simulink model "ABS_discDyn_model"  (R2022b)
settings: Solver=VariableStepAuto  StartTime=0.0  StopTime=tf  MaxStep=1e-3  RelTol=1e-3  EnableMultiTasking=on
values from neighbouring files (symbols this model uses):
  init_speed = 100    [mainABS.m]
  lambda_max = 0.25    [mainABS.m]
  lambda_min = 0.08    [mainABS.m]
  omega_act = 70    [mainABS.m]
  tau_delay = 10e-3    (= 0.01)    [mainABS.m]
  Tb_max = 1400    [mainABS.m]
  Tb_min = 1150    [mainABS.m]
undefined symbols (not defined in the file or in its folder): auxdata
libraries: simulink x1
settings Model: Creator=luca  LastModifiedBy=giacomo
settings SolverCC: AlgebraicLoopSolver=TrustRegion
settings DataIOCC: LimitDataPoints=on  ReturnWorkspaceOutputs=off
settings OptimizationCC: LifeSpan=inf
settings DebuggingCC: UnconnectedInputMsg=warning  UnconnectedOutputMsg=warning  UnconnectedLineMsg=warning  AllowSymbolicDim=off  SFUnexpectedBacktrackingDiag=warning  SFNoUnconditionalDefaultTransitionDiag=warning  SFExecutionAtInitializationDiag=none  SFMachineParentedDataDiag=warning  ArithmeticOperatorsInVariantConditions=warning
settings ModelReferenceCC: EnableRefExpFcnMdlSchedulingChecks=on  PropagateSignalLabelsOutOfModel=off
settings SFSimCC: SimUseLocalCustomCode=off  CustomCodeUndefinedFunction=UseInterfaceOnly
settings RTWCC: RTWUseLocalCustomCode=off
settings CodeAppCC: StateflowObjectComments=on
settings GRTTargetCC: TargetLangStandard=C89/C90 (ANSI)
settings ConfigComp: CovMetricSettings=dw  CovSaveCumulativeToWorkspaceVar=on  CovSaveSingleToWorkspaceVar=on  CovExternalEMLEnable=off

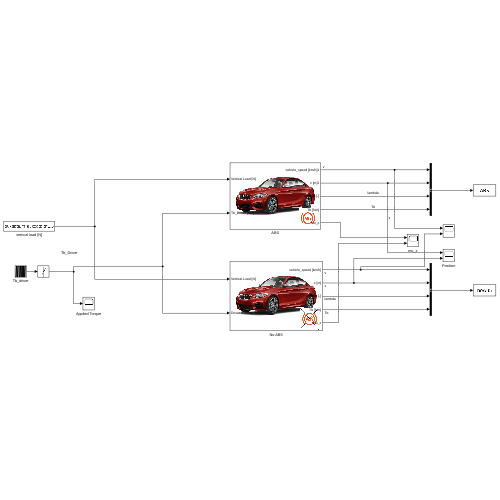
[thumbnail: Simulink's stored preview of the top-level diagram]
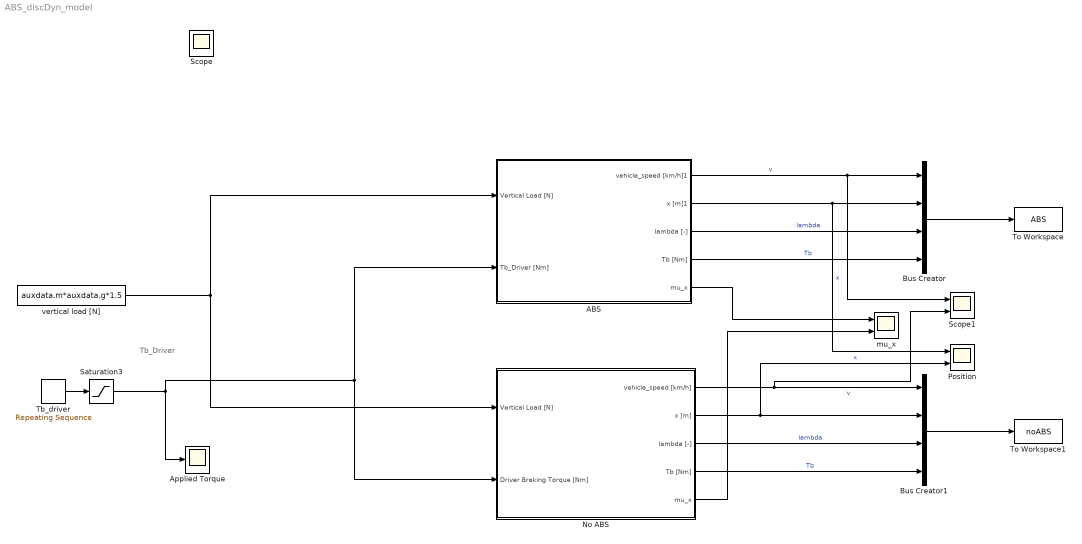
== system ABS_discDyn_model ==
  note: Tb_Driver
  ABS : Subsystem
      mask Display: image('figures/ABScar_on.png');
  Applied Torque : Scope
  Bus Creator : BusCreator  Inputs=4
  Bus Creator1 : BusCreator  Inputs=4
  No ABS : Subsystem
      mask Display: image('figures/ABS_off.png');
  Position : Scope  NumInputPorts=2
  Saturation3 : Saturate  UpperLimit=Tb_max  LowerLimit=0
  Scope1 : Scope  NumInputPorts=2
  Tb_driver : simulink/Sources/Repeating Sequence  rep_seq_t=time_manoeuvre  rep_seq_y=output_manoeuvre
  To Workspace : ToWorkspace  VariableName=ABS  SaveFormat=Timeseries  SampleTime=-1
  To Workspace1 : ToWorkspace  VariableName=noABS  SaveFormat=Timeseries  SampleTime=-1
  mu_x : Scope  NumInputPorts=2
  vertical load [N] : Constant  Value=auxdata.m*auxdata.g*1.5
  Scope : Scope
  wires:
  vertical load [N]/1 -> ABS/1(Vertical Load [N]), No ABS/1(Vertical Load [N])
  No ABS/1(" vehicle_speed [km/h]") -> Scope1/2, Bus Creator1/1  "v"
  No ABS/2(x [m]) -> Position/2, Bus Creator1/2  "x"
  ABS/1(vehicle_speed [km/h]1) -> Scope1/1, Bus Creator/1  "v"
  ABS/2(x [m]1) -> Position/1, Bus Creator/2  "x"
  Bus Creator/1 -> To Workspace/1
  ABS/3(lambda [-]) -> Bus Creator/3  "lambda"
  ABS/4(Tb [Nm]) -> Bus Creator/4  "Tb"
  Bus Creator1/1 -> To Workspace1/1
  No ABS/3(lambda [-]) -> Bus Creator1/3  "lambda"
  No ABS/4(Tb [Nm]) -> Bus Creator1/4  "Tb"
  Saturation3/1 -> ABS/2(Tb_Driver [Nm]), No ABS/2(Driver Braking Torque [Nm]), Applied Torque/1
  Tb_driver/1 -> Saturation3/1
  No ABS/5(mu_x) -> mu_x/2
  ABS/5(mu_x) -> mu_x/1

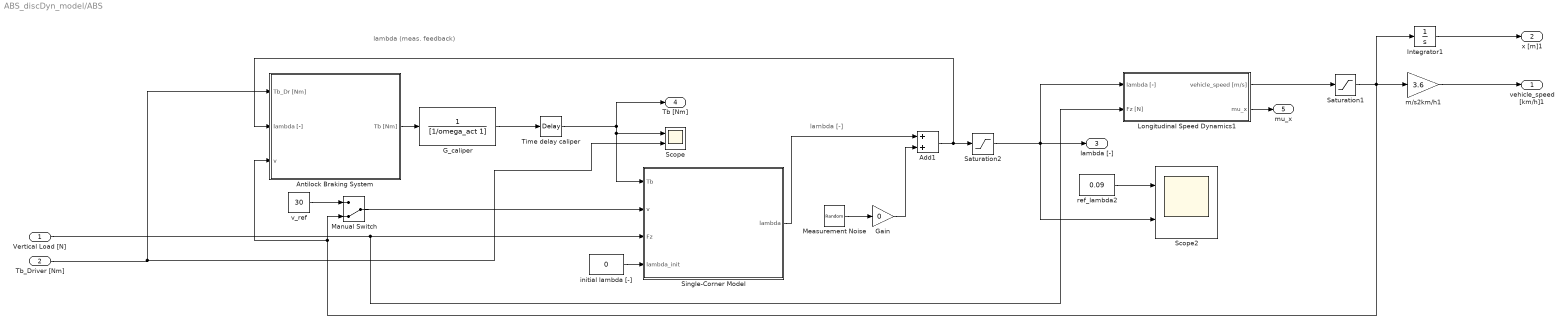
== system ABS_discDyn_model/ABS ==
  note: lambda (meas. feedback)
  note: lambda [-]
  Vertical Load [N] : Inport
  Tb_Driver [Nm] : Inport  Port=2
  Add1 : Sum
  Antilock Braking System : Subsystem
      mask Display: image('figures/ABS_on.png');
  G_caliper : TransferFcn  Numerator=1  Denominator=[1/omega_act 1]
  Gain : Gain  Gain=0
  Integrator1 : Integrator
  Longitudinal Speed Dynamics1 : Subsystem
  Manual Switch : ManualSwitch  CurrentSetting=0
  Measurement Noise : RandomNumber  Variance=2e-5  SampleTime=0.001
  Saturation1 : Saturate  UpperLimit=100  LowerLimit=1e-3
  Saturation2 : Saturate  UpperLimit=1  LowerLimit=0
  Scope : Scope  NumInputPorts=2
  Scope2 : Scope  NumInputPorts=2
  Single-Corner Model : Subsystem
      mask Display:
      | image('figures/caliper_img.jpeg');
      | color('red');
      | port_label('output',1,'lambda');
      | port_label('input',1,'Tb');
      | port_label('input',2,'v');
      | port_label('input',3,'Fz');
      | port_label('input',4,'lambda_init');
  Time delay caliper : TransportDelay  DelayTime=tau_delay
  initial lambda [-] : Constant  Value=0
  m/s2km/h1 : Gain  Gain=3.6
  ref_lambda2 : Constant  Value=0.09
  v_ref : Constant  Value=30
  vehicle_speed [km/h]1 : Outport
  x [m]1 : Outport  Port=2
  lambda [-] : Outport  Port=3
  Tb [Nm] : Outport  Port=4
  mu_x : Outport  Port=5
  wires:
  Add1/1 -> Antilock Braking System/2(lambda [-]), Saturation2/1
  m/s2km/h1/1 -> vehicle_speed [km/h]1/1
  Tb_Driver [Nm]/1 -> Antilock Braking System/1(Tb_Dr [Nm]), Scope/2
  Antilock Braking System/1(Tb [Nm]) -> G_caliper/1
  Saturation2/1 -> lambda [-]/1, Scope2/2, Longitudinal Speed Dynamics1/1(lambda [-])
  Gain/1 -> Add1/2
  initial lambda [-]/1 -> Single-Corner Model/4(lambda_init)
  Longitudinal Speed Dynamics1/1(vehicle_speed [m/s]) -> Saturation1/1
  Integrator1/1 -> x [m]1/1
  Single-Corner Model/1(lambda) -> Add1/1
  Vertical Load [N]/1 -> Single-Corner Model/3(Fz), Longitudinal Speed Dynamics1/2(Fz [N])
  ref_lambda2/1 -> Scope2/1
  Measurement Noise/1 -> Gain/1
  Saturation1/1 -> Antilock Braking System/3(v), Manual Switch/2, Integrator1/1, m/s2km/h1/1
  Manual Switch/1 -> Single-Corner Model/2(v)
  v_ref/1 -> Manual Switch/1
  Longitudinal Speed Dynamics1/2(mu_x) -> mu_x/1
  G_caliper/1 -> Time delay caliper/1
  Time delay caliper/1 -> Tb [Nm]/1, Single-Corner Model/1(Tb), Scope/1

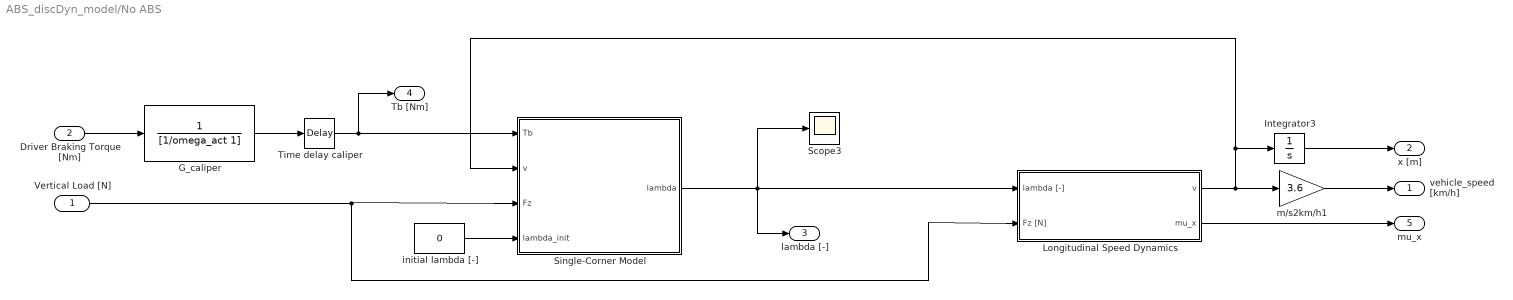
== system ABS_discDyn_model/No ABS ==
  Vertical Load [N] : Inport
  Driver Braking Torque [Nm] : Inport  Port=2
  G_caliper : TransferFcn  Numerator=1  Denominator=[1/omega_act 1]
  Integrator3 : Integrator
  Longitudinal Speed Dynamics : Subsystem
  Scope3 : Scope
  Single-Corner Model : Subsystem
      mask Display:
      | image('figures/caliper_img.jpeg');
      | color('red');
      | port_label('output',1,'lambda [-]');
      | port_label('input',1,'Tb [Nm]');
      | port_label('input',2,'v [m/s]');
      | port_label('input',3,'Fz [N]');
      | port_label('input',4,'lambda_init [-]');
  Time delay caliper : TransportDelay  DelayTime=tau_delay
  initial lambda [-] : Constant  Value=0
  m/s2km/h1 : Gain  Gain=3.6
  " vehicle_speed [km/h]" : Outport
  x [m] : Outport  Port=2
  lambda [-] : Outport  Port=3
  Tb [Nm] : Outport  Port=4
  mu_x : Outport  Port=5
  wires:
  Single-Corner Model/1(lambda) -> lambda [-]/1, Longitudinal Speed Dynamics/1(lambda [-]), Scope3/1
  Vertical Load [N]/1 -> Single-Corner Model/3(Fz), Longitudinal Speed Dynamics/2(Fz [N])
  Time delay caliper/1 -> Tb [Nm]/1, Single-Corner Model/1(Tb)
  initial lambda [-]/1 -> Single-Corner Model/4(lambda_init)
  m/s2km/h1/1 -> " vehicle_speed [km/h]"/1
  Integrator3/1 -> x [m]/1
  Longitudinal Speed Dynamics/1(v) -> Single-Corner Model/2(v), Integrator3/1, m/s2km/h1/1
  Longitudinal Speed Dynamics/2(mu_x) -> mu_x/1
  G_caliper/1 -> Time delay caliper/1
  Driver Braking Torque [Nm]/1 -> G_caliper/1

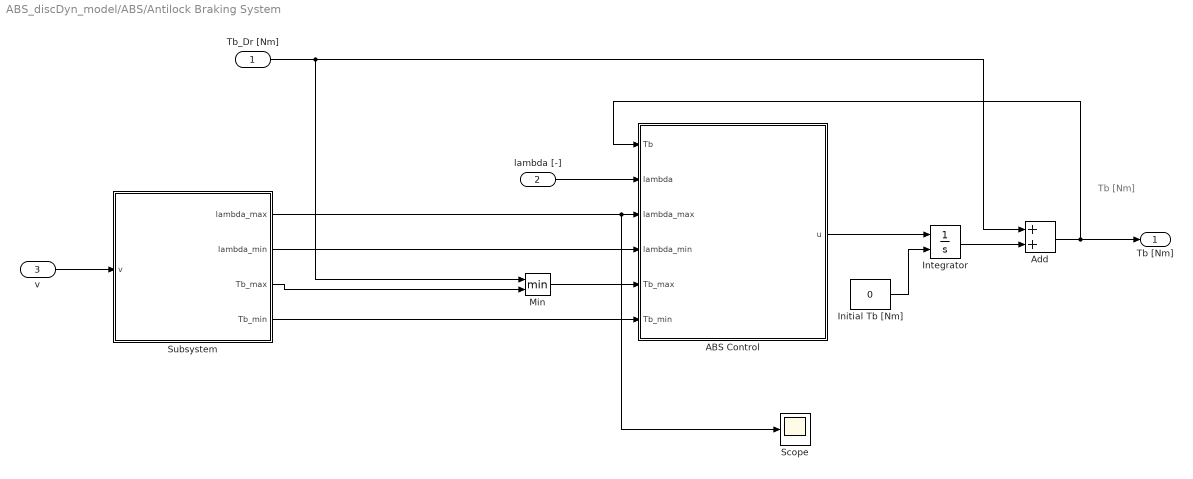
== system ABS_discDyn_model/ABS/Antilock Braking System ==
  note: Tb [Nm]
  Tb_Dr [Nm] : Inport
  lambda [-] : Inport  Port=2
  v : Inport  Port=3
  ABS Control : Stateflow chart  TreatAsAtomicUnit=on
  Add : Sum
  Initial Tb [Nm] : Constant  Value=0
  Integrator : Integrator  InitialConditionSource=external
  Min : MinMax  Inputs=2
  Scope : Scope
  Subsystem : Subsystem
  Tb [Nm] : Outport
  wires:
  lambda [-]/1 -> ABS Control/2(lambda)
  Initial Tb [Nm]/1 -> Integrator/2
  Add/1 -> ABS Control/1(Tb), Tb [Nm]/1
  ABS Control/1(u) -> Integrator/1
  Integrator/1 -> Add/2
  Tb_Dr [Nm]/1 -> Min/1, Add/1
  Subsystem/1(lambda_max) -> Scope/1, ABS Control/3(lambda_max)
  v/1 -> Subsystem/1(v)
  Subsystem/4(Tb_min) -> ABS Control/6(Tb_min)
  Subsystem/2(lambda_min) -> ABS Control/4(lambda_min)
  Min/1 -> ABS Control/5(Tb_max)
  Subsystem/3(Tb_max) -> Min/2

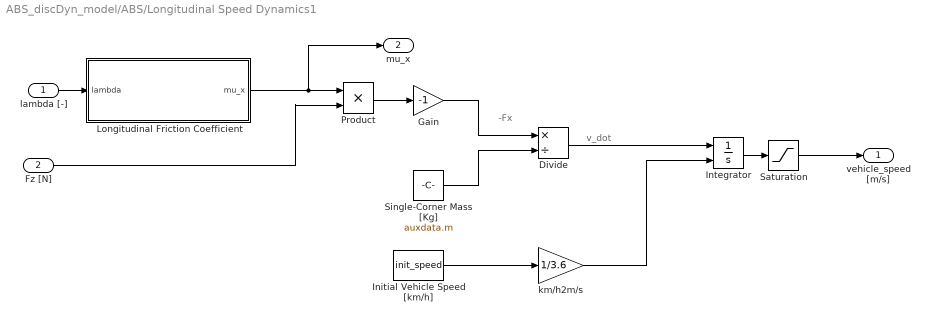
== system ABS_discDyn_model/ABS/Longitudinal Speed Dynamics1 ==
  note: -Fx
  note: v_dot
  lambda [-] : Inport
  Fz [N] : Inport  Port=2
  Divide : Product  Inputs=*/
  Gain : Gain  Gain=-1
  Initial Vehicle Speed [km/h] : Constant  Value=init_speed
  Integrator : Integrator  InitialConditionSource=external
  Longitudinal Friction Coefficient : MATLAB Function  TreatAsAtomicUnit=on
  Product : Product
  Saturation : Saturate  UpperLimit=100  LowerLimit=0
  Single-Corner Mass [Kg] : Constant  Value=auxdata.m
  km/h2m/s : Gain  Gain=1/3.6
  vehicle_speed [m/s] : Outport
  mu_x : Outport  Port=2
  wires:
  Single-Corner Mass [Kg]/1 -> Divide/2
  Divide/1 -> Integrator/1
  km/h2m/s/1 -> Integrator/2
  Initial Vehicle Speed [km/h]/1 -> km/h2m/s/1
  Product/1 -> Gain/1
  Gain/1 -> Divide/1
  Saturation/1 -> vehicle_speed [m/s]/1
  Integrator/1 -> Saturation/1
  Longitudinal Friction Coefficient/1(mu_x) -> mu_x/1, Product/1
  Fz [N]/1 -> Product/2
  lambda [-]/1 -> Longitudinal Friction Coefficient/1(lambda)

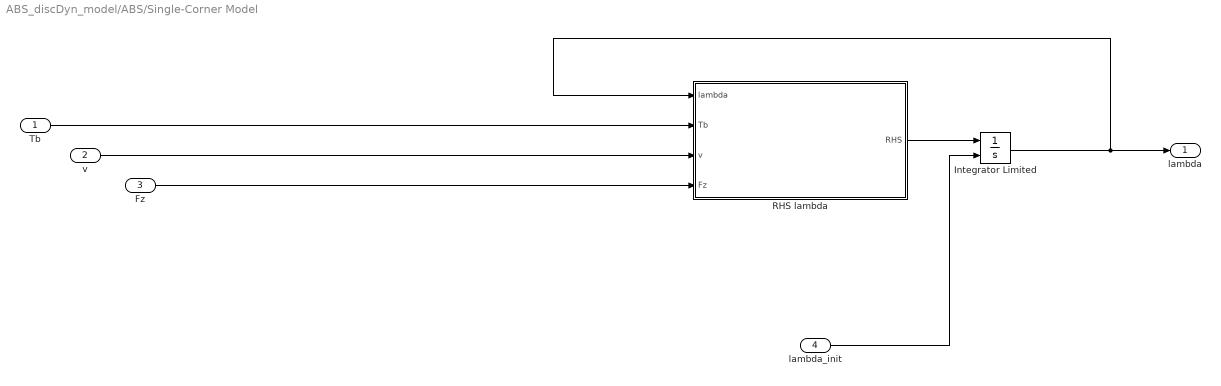
== system ABS_discDyn_model/ABS/Single-Corner Model ==
  Tb : Inport
  v : Inport  Port=2
  Fz : Inport  Port=3
  lambda_init : Inport  Port=4
  Integrator Limited : Integrator  InitialConditionSource=external  LimitOutput=on  UpperSaturationLimit=0.99  LowerSaturationLimit=0
  RHS lambda : MATLAB Function  TreatAsAtomicUnit=on
  lambda : Outport
  wires:
  lambda_init/1 -> Integrator Limited/2
  RHS lambda/1(RHS) -> Integrator Limited/1
  v/1 -> RHS lambda/3(v)
  Fz/1 -> RHS lambda/4(Fz)
  Integrator Limited/1 -> RHS lambda/1(lambda), lambda/1
  Tb/1 -> RHS lambda/2(Tb)

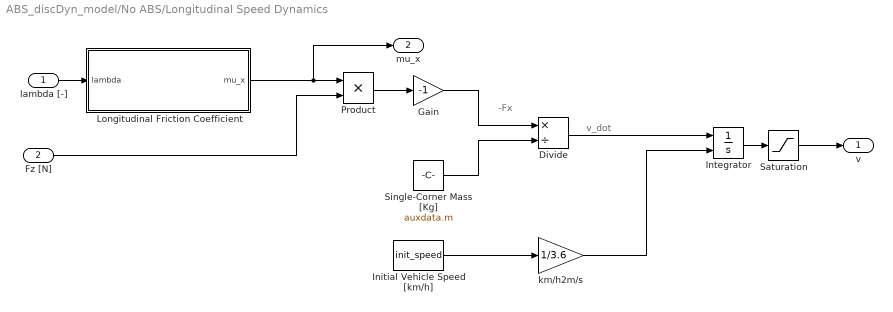
== system ABS_discDyn_model/No ABS/Longitudinal Speed Dynamics ==
  note: -Fx
  note: v_dot
  lambda [-] : Inport
  Fz [N] : Inport  Port=2
  Divide : Product  Inputs=*/
  Gain : Gain  Gain=-1
  Initial Vehicle Speed [km/h] : Constant  Value=init_speed
  Integrator : Integrator  InitialConditionSource=external
  Longitudinal Friction Coefficient : MATLAB Function  TreatAsAtomicUnit=on
  Product : Product
  Saturation : Saturate  UpperLimit=100  LowerLimit=1e-3
  Single-Corner Mass [Kg] : Constant  Value=auxdata.m
  km/h2m/s : Gain  Gain=1/3.6
  v : Outport
  mu_x : Outport  Port=2
  wires:
  Single-Corner Mass [Kg]/1 -> Divide/2
  Divide/1 -> Integrator/1
  km/h2m/s/1 -> Integrator/2
  Initial Vehicle Speed [km/h]/1 -> km/h2m/s/1
  Product/1 -> Gain/1
  Gain/1 -> Divide/1
  Saturation/1 -> v/1
  Integrator/1 -> Saturation/1
  Longitudinal Friction Coefficient/1(mu_x) -> mu_x/1, Product/1
  Fz [N]/1 -> Product/2
  lambda [-]/1 -> Longitudinal Friction Coefficient/1(lambda)

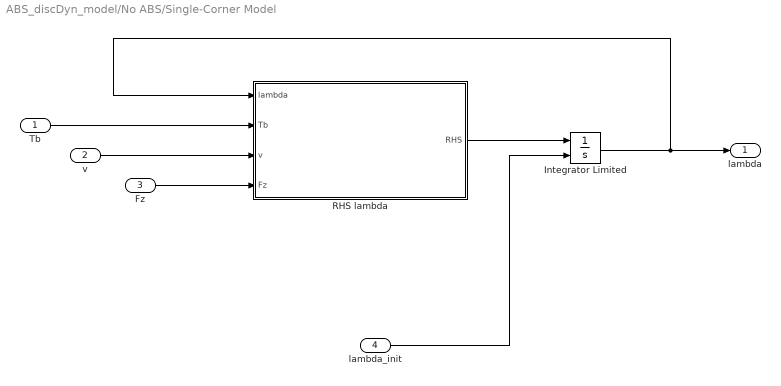
== system ABS_discDyn_model/No ABS/Single-Corner Model ==
  Tb : Inport
  v : Inport  Port=2
  Fz : Inport  Port=3
  lambda_init : Inport  Port=4
  Integrator Limited : Integrator  InitialConditionSource=external  LimitOutput=on  UpperSaturationLimit=0.99  LowerSaturationLimit=0
  RHS lambda : MATLAB Function  TreatAsAtomicUnit=on
  lambda : Outport
  wires:
  Tb/1 -> RHS lambda/2(Tb)
  lambda_init/1 -> Integrator Limited/2
  RHS lambda/1(RHS) -> Integrator Limited/1
  v/1 -> RHS lambda/3(v)
  Fz/1 -> RHS lambda/4(Fz)
  Integrator Limited/1 -> RHS lambda/1(lambda), lambda/1

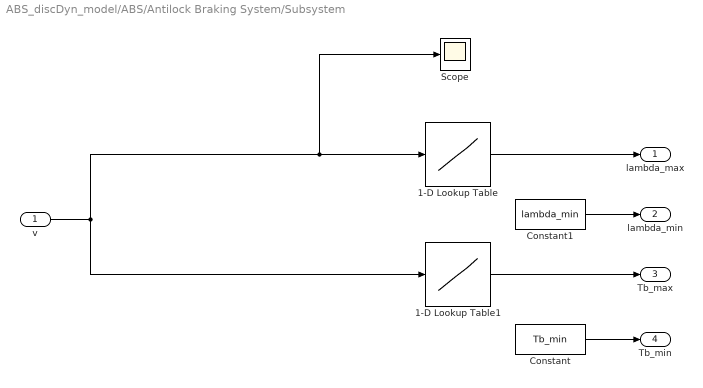
== system ABS_discDyn_model/ABS/Antilock Braking System/Subsystem ==
  v : Inport
  1-D Lookup Table : Lookup_n-D  NumberOfTableDimensions=1  BreakpointsForDimension1=[5;30]  Table=[0.1;lambda_max]  ExtrapMethod=Clip  InternalRulePriority=Speed  RndMeth=Simplest
  1-D Lookup Table1 : Lookup_n-D  NumberOfTableDimensions=1  BreakpointsForDimension1=[5;30]  Table=[1250;1400]  ExtrapMethod=Clip  InternalRulePriority=Speed  RndMeth=Simplest
  Constant : Constant  Value=Tb_min
  Constant1 : Constant  Value=lambda_min
  Scope : Scope
  lambda_max : Outport
  lambda_min : Outport  Port=2
  Tb_max : Outport  Port=3
  Tb_min : Outport  Port=4
  wires:
  Constant/1 -> Tb_min/1
  Constant1/1 -> lambda_min/1
  v/1 -> 1-D Lookup Table1/1, Scope/1, 1-D Lookup Table/1
  1-D Lookup Table/1 -> lambda_max/1
  1-D Lookup Table1/1 -> Tb_max/1

== matlab function ABS_discDyn_model/No ABS/Single-Corner Model/RHS lambda ==
  data: lambda input; RHS output; Tb input; v input; Fz input; auxdata parameter
function RHS = lambdaDyn( lambda, Tb, v, Fz, auxdata )
% Right hand side of the longitudinal slip dynamics

omega = (1 - lambda) * v / auxdata.r_w + eps;

% Equilibrium manifold
%        /      (1 - lambda) * J \
% Psi = | r_w + ----------------  | * Fz * mu
%        \          r_w * m      /
Psi = (auxdata.r_w + ((1 - lambda) .* auxdata.J) / ...
      (auxdata.r_w * auxdata.m)) .* Fz .* burckhardt( lambda, 'Dry Asphalt' );

RHS = -(1 - lambda) / (auxdata.J * omega) * (Psi - Tb);

end

== stateflow chart ABS_discDyn_model/ABS/Antilock Braking System/ABS Control ==
  state ABS_ON
    state State_q3
      entry: u = 0;
    state State_q2
      entry: u = -k;
    state State_q0
      entry: u = k;
    state State_q1
      entry: u = 0;
    State_q2 -> State_q3 : [Tb <= Tb_min]
    State_q3 -> State_q0 : [lambda <= lambda_min]
    (default) -> State_q0
    State_q1 -> State_q2 : [lambda >= lambda_max]
    State_q0 -> State_q1 : [Tb >= Tb_max]
  (default) -> ABS_ON
  data: Tb input; k parameter; lambda input; u output; lambda_max input; lambda_min input; Tb_max input; Tb_min input

== matlab function ABS_discDyn_model/No ABS/Longitudinal Speed Dynamics/Longitudinal Friction Coefficient ==
  data: lambda input; mu_x output; auxdata parameter
function mu_x = LongitudinalFrction( lambda, auxdata )
    
mu_x = burckhardt( lambda, auxdata.road_condition );

end

== matlab function ABS_discDyn_model/ABS/Longitudinal Speed Dynamics1/Longitudinal Friction Coefficient ==
  data: lambda input; mu_x output; auxdata parameter
function mu_x = LongitudinalFrction(lambda,auxdata)
    
mu_x = burckhardt(lambda,auxdata.road_condition);

end

== matlab function ABS_discDyn_model/ABS/Single-Corner Model/RHS lambda ==
  data: lambda input; RHS output; Tb input; v input; Fz input; auxdata parameter
function RHS = lambdaDyn( lambda, Tb, v, Fz, auxdata )
% Right hand side of the longitudinal slip dynamics

omega = (1 - lambda) * v / auxdata.r_w;

% Equilibrium manifold
%        /      (1 - lambda) * J \
% Psi = | r_w + ----------------  | * Fz * mu
%        \          r_w * m      /
Psi = (auxdata.r_w + ...
       auxdata.J / (auxdata.r_w * auxdata.m) * (1 - lambda)) * Fz * ...
       burckhardt( lambda, auxdata.road_condition );

if omega <= 0.1
    RHS = 0;
else
    RHS = -(1 - lambda) / (auxdata.J * omega) * (Psi - Tb);
end

end
